simulink model "task7_lab12"  (R2021a)
settings: Solver=VariableStepAuto  StartTime=0.0  StopTime=20  RelTol=1e-3
settings Model: Creator=reemb  LastModifiedBy=reemb

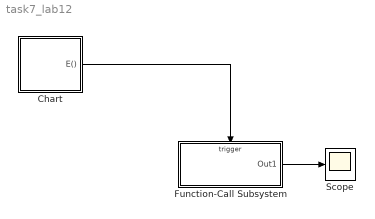
== system task7_lab12 ==
  Chart : Stateflow chart  TreatAsAtomicUnit=on
  Function-Call Subsystem : Subsystem  TreatAsAtomicUnit=on
  Scope : Scope
  wires:
  Function-Call Subsystem/1(Out1) -> Scope/1
  Chart/1(E()) -> Function-Call Subsystem/Trigger

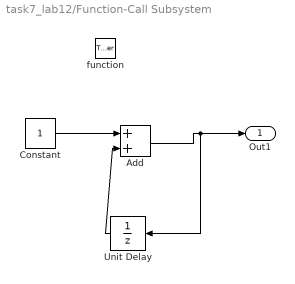
== system task7_lab12/Function-Call Subsystem ==
  function : TriggerPort  TriggerType=function-call  VariantControl=(inherit)  StatesWhenEnabling=reset
  Add : Sum
  Constant : Constant
  Unit Delay : UnitDelay  SampleTime=-1  HasFrameUpgradeWarning=on
  Out1 : Outport
  wires:
  Unit Delay/1 -> Add/2
  Add/1 -> Unit Delay/1, Out1/1
  Constant/1 -> Add/1

== stateflow chart task7_lab12/Chart ==
  settings: updateMethod=DISCRETE  sampleTime=0.1
  state ON
    during: E;
  state OFF
  ON -> OFF : after(5, sec)
  (default) -> ON
  OFF -> ON : after(5, sec)
  events: E output FUNCTION_CALL_EVENT
